simulink model "AdaptiveIDMF"  (R2022a)
settings: Solver=ode4  StartTime=0.0  StopTime=30  FixedStep=0.01  RelTol=1e-3
PostLoadFcn:
  | %Add subfolders to path
  | addpath('virtualworld');
InitFcn:
  | startScript;
values from neighbouring files (symbols this model uses):
  angularVelocity = [0 0 -0.01]    [startScript.m]
  angularVelocityforLanding = [0 0 0]    [startScript.m]
  dronestartlocation = [-1.5 0 4]    [startScript.m]
  Dstar = -0.5    [startScript.m]
  finalHoverHeight = 2.5    [startScript.m]
  helipadLocation = [14 0.6 5]    [startScript.m]
  linearVelocity = [5 0.05 1]    [startScript.m]
  linearVelocityforHover = [0.65 0.05 0.3]    [startScript.m]
  ypmin = yps(iypmin,:)    [hyperpred.m]
undefined symbols (not defined in the file or in its folder): fspecial, gcbh, Kanade, Lucas, Rec, SDTV, vrmfunc
libraries: visiontextngfix x10, visionconversions x9, vrlib x7, visionanalysis x7, slpidlib x4, sharedtransform x2, simulink x1
(part 3 of 3)

== matlab function AdaptiveIDMF/ Optical Flow Algorithm for Obstacle Avoidance/Subsystem/MATLAB Function1 ==
  settings: updateMethod=DISCRETE  sampleTime=0.01
  data: videoFrameGray input; newFeaturePointLocations output size=[50 2]; featurePointLocations input; numberOfFeaturePoints output; Reset output; oldInliers output size=[50 2]; noofpoints input
% Function for tracking face and feature points
%
% Copyright 2016 The MathWorks, Inc.
function [newFeaturePointLocations, numberOfFeaturePoints,Reset, oldInliers]   = trackPoints(videoFrameGray, featurePointLocations,noofpoints)

persistent pointTracker
persistent oldPoints
% persistent bboxPoints
persistent first_time
persistent numPts
% persistent vel_lines
% persistent N
reset = 0;
x=0;
x1=single(zeros(50,2));
% Create the point tracker object.
if isempty(pointTracker)
    pointTracker = vision.PointTracker('MaxBidirectionalError', 10,'MaxIterations',50);
end
% 
% if isempty(bboxPoints)
%     bboxPoints = [0 0];
% end 

if isempty(oldPoints)
    oldPoints = single(zeros(50,2));
end      

if isempty(numPts)
    numPts = 0;
end

% if isempty(N)
%     N = 0;
% end
% 
% if isempty(vel_lines)
%     vel_lines = single(zeros(25,4));
% end

if isempty (reset)
    reset=0;
end

% Initialize tracker with dummy points
if isempty(first_time)
   initialize(pointTracker, single([10 10]),videoFrameGray);
   first_time = 0;
end

if numPts ==0 
    if featurePointLocations~=single(zeros(50,2))
        % Re-initialize the point tracker if a face has been detected and
        % feature points obtained.
        newFeaturePointLocations = featurePointLocations;
        numPts = size(newFeaturePointLocations,1);
        
        if ~pointTracker.isLocked
            initialize(pointTracker, newFeaturePointLocations,videoFrameGray);
        end
 
        %step(pointTracker, videoFrameGray);
        setPoints(pointTracker, newFeaturePointLocations);
        
        % Save a copy of the points.
        oldPoints = newFeaturePointLocations;
        oldInliers = oldPoints;
        % Convert the rectangle represented as [x, y, w, h] into an
        % M-by-2 matrix of [x,y] coordinates of the four corners. This
        % is needed to be able to transform the bounding box to display
        % the orientation of the face.
%         bboxPoints = bbox2points(bBox(1, :));
%         bBoxCornerPts = bboxPoints;
    else
%         bBoxCornerPts = [];
        newFeaturePointLocations = single(zeros(25,2));
        numPts=0;
        oldInliers = single(zeros(25,2));
    end

else
    % Tracking mode. 
    [newFeaturePointLocations, isFound] = step(pointTracker, videoFrameGray);
    assert(size(newFeaturePointLocations, 1) < 500);
    visiblePoints = newFeaturePointLocations(isFound, :);
    oldInliers = oldPoints(isFound, :);
    numPts = size(oldInliers,1);
    numPts1 = size(visiblePoints, 1);

    if numPts1>noofpoints && numPts>=noofpoints
        %       if numPts1>=45 abs(numPts1 -numPts) <= 5
        % Estimate the geometric transformation between the old points
        % and the new points.
%         [xform, inlierIdx] = estimateGeometricTransform2D(...
%             oldInliers, visiblePoints, 'similarity', 'MaxDistance', 20);
%         visiblePoints = visiblePoints(inlierIdx, :);

%         % Apply the transformation to the bounding box.
%         bboxPoints = double(transformPointsForward(xform, bboxPoints));
%         bBoxCornerPts = bboxPoints;

        % Assign the visible feature points
        assert(size(visiblePoints, 1) < 500);
        newFeaturePointLocations = visiblePoints;
        numPts=size(newFeaturePointLocations,1);

        % Reset the points.
        oldPoints = visiblePoints;
        setPoints(pointTracker, oldPoints);
    else
%         bBoxCornerPts = [];
%         newFeaturePointLocations = single([]);  
%         numPts=0;
        reset =1 ;
        if featurePointLocations~=single(zeros(50,2))
            % Re-initialize the point tracker if a face has been detected and
            % feature points obtained.
            % 480x320

%             x1=featurePointLocations(:,1)>100 & featurePointLocations(:,1)<380;
%             newFeaturePointLocations=featurePointLocations(x1,:);
%             
%             y1=newFeaturePointLocations(:,2)>80 & newFeaturePointLocations(:,2)<240;
%             newFeaturePointLocations=newFeaturePointLocations(y1,:);

            newFeaturePointLocations=featurePointLocations;
%             newFeaturePointLocations = padarray(featurePointLocations,50-length(featurePointLocations),0,'post');
%             numPts = size(newFeaturePointLocations,1)
            
            if ~pointTracker.isLocked
            initialize(pointTracker, newFeaturePointLocations,videoFrameGray);
            end  

            step(pointTracker, videoFrameGray);
            numPts = size(newFeaturePointLocations,1);
            setPoints(pointTracker, newFeaturePointLocations);
            
            % Save a copy of the points.
            oldPoints = newFeaturePointLocations;
            oldInliers = oldPoints;

        else

            newFeaturePointLocations = single(zeros(25,2));
            numPts=0;

        end

    end

end

numberOfFeaturePoints = numPts;
Reset=reset;

== matlab function AdaptiveIDMF/ Optical Flow Algorithm for Obstacle Avoidance/Subsystem/D_cap/sumele ==
  data: u input; y1 output; n1 output
function [y1,n1] = fcn(u)
u1=rmoutliers(u);
u2=rmoutliers(u,'percentiles',[30 70]);
n1=length(u1);
n2=length(u2);
% if n1==1
%     y1=0.00;
% else
y1 = double(sum(u1));
% end
y2 = double(sum(u2));
if n2==1
    y2=0.00;
else
y2 = double(sum(u2))/n2;
end

== matlab function AdaptiveIDMF/ Optical Flow Algorithm for Obstacle Avoidance/Subsystem/Length of line ==
  data: lines input; oldlines input; l1 output size=5000; l2 output size=5000; N output
function [l1,l2,N] = fcn(lines,oldlines)
l1=single([]);
l2=single([]);
% persistent x;
% % size(x)
% if isempty(x)
%     x=lines;
% end
% if reset>0
%     oldlines=x;
% else
%     oldlines=lines;
% end
N = 0;
% % size(lines)
% if isempty(nonzeros(oldlines))
%     oldlines=lines;
% end

a1=size(lines);
a1=a1(1,1);
a2=size(oldlines);
a2=a2(1,1);
lines = sortrows(lines);
oldlines=sortrows(oldlines);
% a1=length(lines);
% a2=length(oldlines);
if a1<=a2
for i = 1: a1
    for j = i:a2
        if abs(lines(i,1) + lines(i,3) - oldlines(j,3) -oldlines(j,1))<=7 && N~=i
           if norm(lines(i,1:2)-lines(i,3:4))~=0 && norm(oldlines(j,1:2)-oldlines(j,3:4))~=0 ...
%                    && norm(lines(i,1:2)-lines(i,3:4))>=norm(oldlines(j,1:2)-oldlines(j,3:4))
            l1 = [l1 ;norm(lines(i,1:2)-lines(i,3:4))];
            l2 = [l2; norm(oldlines(j,1:2)-oldlines(j,3:4))];
            N = N+1;
           end
        end
    end
end
else
for i = 1: a2
    for j = i:a1
        if abs(oldlines(i,1) + oldlines(i,3) - lines(j,3) -lines(j,1))<=7  && N~=i
           if norm(lines(j,1:2)-lines(j,3:4))~=0 && norm(oldlines(i,1:2)-oldlines(i,3:4))~=0 ...
%                    && norm(lines(j,1:2)-lines(j,3:4))>=norm(oldlines(i,1:2)-oldlines(i,3:4))
            l1 = [l1 ;norm(lines(j,1:2)-lines(j,3:4))];
            l2 = [l2; norm(oldlines(i,1:2)-oldlines(i,3:4))];
            N = N+1;
           end
        end
    end
end
end
x=lines;

== matlab function AdaptiveIDMF/ Optical Flow Algorithm for Obstacle Avoidance/Subsystem/Points to Line ==
  data: newpoints input; New_Lines output size=[2000,4]; oldpoints input; Old_Lines output size=[2000,4]
function [New_Lines, Old_Lines] = fcn(newpoints,oldpoints)


rop=round(newpoints*100)/100;
rop1=round(oldpoints*100)/100;

X = [];
Y = [];
shiftX = [];
shiftY=[];
X1 = [];
Y1 = [];
shiftX1 = [];
shiftY1=[];
%(orderedpoints(i,1)==orderedpoints(i+1,1)|| orderedpoints(i,1)==orderedpoints(i+1,1)+1 || orderedpoints(i,1)==orderedpoints(i+1,1)-1 ...
                %|| orderedpoints(i,1)==orderedpoints(i+1,1)+2 || orderedpoints(i,1)==orderedpoints(i+1,1)-2) &&
%|| orderedpoints(i,1)==orderedpoints(i+1,1)+1 || orderedpoints(i,1)==orderedpoints(i+1,1)-1)


% if length(orderedpoints)>2
% for i = 1:2:length(orderedpoints)-1
%     if i ==1 && orderedpoints(i,1)==orderedpoints(i+1,1)
%         X = [X ;orderedpoints(i,1)];
%         Y = [Y ;orderedpoints(i,2)];
%         shiftX = [shiftX ;orderedpoints(i+1,1)];
%         shiftY = [shiftY ;orderedpoints(i+1,2)];
% 
%         X1 = [X1 ;orderedpoints1(i,1)];
%         Y1 = [Y1 ;orderedpoints1(i,2)];
%         shiftX1 = [shiftX1 ;orderedpoints1(i+1,1)];
%         shiftY1 = [shiftY1 ;orderedpoints1(i+1,2)];
%     else
%         if i ~=1 && (abs(orderedpoints(i,1)-orderedpoints(i+1,1))<3)
%         X = [X ;orderedpoints(i,1)];
%         Y = [Y ;orderedpoints(i,2)];
%         shiftX = [shiftX ;orderedpoints(i+1,1)];
%         shiftY = [shiftY ;orderedpoints(i+1,2)];
% 
%         X1 = [X1 ;orderedpoints1(i,1)];
%         Y1 = [Y1 ;orderedpoints1(i,2)];
%         shiftX1 = [shiftX1 ;orderedpoints1(i+1,1)];
%         shiftY1 = [shiftY1 ;orderedpoints1(i+1,2)];
%         
%         elseif i~=1 &&  (abs(orderedpoints(i,1)-orderedpoints(i-1,1))<2)
%         X = [X ;orderedpoints(i,1)];
%         Y = [Y ;orderedpoints(i,2)];
%         shiftX = [shiftX ;orderedpoints(i-1,1)];
%         shiftY = [shiftY ;orderedpoints(i-1,2)];
% 
%         X1 = [X1 ;orderedpoints1(i,1)];
%         Y1 = [Y1 ;orderedpoints1(i,2)];
%         shiftX1 = [shiftX1 ;orderedpoints1(i-1,1)];
%         shiftY1 = [shiftY1 ;orderedpoints1(i-1,2)];
%     end
%     end
% end
% for i = 1:2:length(orderedpoints2)-1
%     if i ==1 && orderedpoints2(i,2)==orderedpoints2(i+1,2)
%         X = [X ;orderedpoints2(i,1)];
%         Y = [Y ;orderedpoints2(i,2)];
%         shiftX = [shiftX ;orderedpoints2(i+1,1)];
%         shiftY = [shiftY ;orderedpoints2(i+1,2)];
% 
%         X1 = [X1 ;orderedpoints3(i,1)];
%         Y1 = [Y1 ;orderedpoints3(i,2)];
%         shiftX1 = [shiftX1 ;orderedpoints3(i+1,1)];
%         shiftY1 = [shiftY1 ;orderedpoints3(i+1,2)];
% 
%     else
%         if i ~=1 && (abs(orderedpoints2(i,2)-orderedpoints2(i+1,2))<3)
%         X = [X ;orderedpoints2(i,1)];
%         Y = [Y ;orderedpoints2(i,2)];
%         shiftX = [shiftX ;orderedpoints2(i+1,1)];
%         shiftY = [shiftY ;orderedpoints2(i+1,2)];
% 
%         X1 = [X1 ;orderedpoints3(i,1)];
%         Y1 = [Y1 ;orderedpoints3(i,2)];
%         shiftX1 = [shiftX1 ;orderedpoints3(i+1,1)];
%         shiftY1 = [shiftY1 ;orderedpoints3(i+1,2)];
%         
%         elseif i~=1 &&  (abs(orderedpoints2(i,2)-orderedpoints2(i-1,2))<2)
%         X = [X ;orderedpoints2(i,1)];
%         Y = [Y ;orderedpoints2(i,2)];
%         shiftX = [shiftX ;orderedpoints2(i-1,1)];
%         shiftY = [shiftY ;orderedpoints2(i-1,2)];
% 
%         X1 = [X1 ;orderedpoints3(i,1)];
%         Y1 = [Y1 ;orderedpoints3(i,2)];
%         shiftX1 = [shiftX1 ;orderedpoints3(i-1,1)];
%         shiftY1 = [shiftY1 ;orderedpoints3(i-1,2)];
%     end
%     end
% end
% % for i = 1:length(orderedpoints)-1
% %     for j=i+1:length(orderedpoints)
% %         X = [X ;orderedpoints(i,1)];
% %         Y = [Y ;orderedpoints(i,2)];
% %         shiftX = [shiftX ;orderedpoints(j,1)];
% %         shiftY = [shiftY ;orderedpoints(j,2)];
% %     end
% % end
% 
%     vel_points = [X(:), Y(:); shiftX(:),  shiftY(:) ];
%     x= single([X(:), Y(:), shiftX(:),  shiftY(:)]);
% 
%     vel_points1 = [X1(:), Y1(:); shiftX1(:),  shiftY1(:) ];
%     x1= single([X1(:), Y1(:), shiftX1(:),  shiftY1(:)]);
% else
%     vel_points = [newpoints; newpoints];
%     x= single([newpoints, newpoints]);
% 
%     vel_points1 = [oldpoints; oldpoints];
%     x1= single([oldpoints, oldpoints]);
% end

for i = 1:length(newpoints)
    for j= i+1:length(newpoints)
        if abs(newpoints(i,1)-newpoints(j,1))<1
            X = [X ;newpoints(i,1)];
            Y = [Y ;newpoints(i,2)];
            shiftX = [shiftX ;newpoints(j,1)];
            shiftY = [shiftY ;newpoints(j,2)];

            X1 = [X1 ;oldpoints(i,1)];
            Y1 = [Y1 ;oldpoints(i,2)];
            shiftX1 = [shiftX1 ;oldpoints(j,1)];
            shiftY1 = [shiftY1 ;oldpoints(j,2)];
        end
    end
end

for i = 1:length(newpoints)
    for j= i+1:length(newpoints)
        if abs(newpoints(i,2)-newpoints(j,2))<2
            X = [X ;newpoints(i,1)];
            Y = [Y ;newpoints(i,2)];
            shiftX = [shiftX ;newpoints(j,1)];
            shiftY = [shiftY ;newpoints(j,2)];

            X1 = [X1 ;oldpoints(i,1)];
            Y1 = [Y1 ;oldpoints(i,2)];
            shiftX1 = [shiftX1 ;oldpoints(j,1)];
            shiftY1 = [shiftY1 ;oldpoints(j,2)];
        end
    end
end
New_Lines=single([X(:), Y(:), shiftX(:),  shiftY(:)]);
Old_Lines=single([X1(:), Y1(:), shiftX1(:),  shiftY1(:)]);
